simulink model "Spring2_Mass2_Damper2"  (R2019a)
settings: Solver=VariableStepAuto  StartTime=0.0  StopTime=100  RelTol=1e-3
values from neighbouring files (symbols this model uses):
  C1 = 1    [value.m]
  C2 = 1    [value.m]
  K1 = 1    [value.m]
  K2 = 1    [value.m]
  M1 = 1    [value.m]
  M2 = 1    [value.m]
settings Model: Creator=Takumi SHIOTA  LastModifiedBy=TakumiShiota

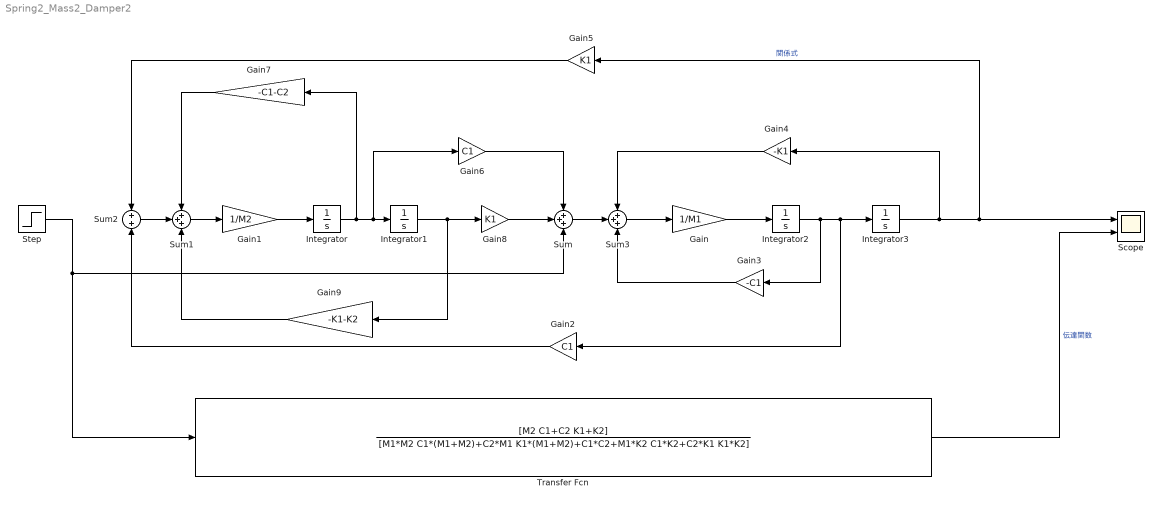
== system Spring2_Mass2_Damper2 ==
  Gain : Gain  Gain=1/M1
  Gain1 : Gain  Gain=1/M2
  Gain2 : Gain  Gain=C1
  Gain3 : Gain  Gain=-C1
  Gain4 : Gain  Gain=-K1
  Gain5 : Gain  Gain=K1
  Gain6 : Gain  Gain=C1
  Gain7 : Gain  Gain=-C1-C2
  Gain8 : Gain  Gain=K1
  Gain9 : Gain  Gain=-K1-K2
  Integrator{,1..3} (4 alike) : Integrator
  Scope : Scope  NumInputPorts=2
  Step : Step  SampleTime=0.0002
  Sum : Sum  Inputs=+++
  Sum1 : Sum  Inputs=+++
  Sum2 : Sum  Inputs=+|+
  Sum3 : Sum  Inputs=+++
  Transfer Fcn : TransferFcn  Numerator=[M2 C1+C2 K1+K2]  Denominator=[M1*M2 C1*(M1+M2)+C2*M1 K1*(M1+M2)+C1*C2+M1*K2 C1*K2+C2*K1 K1*K2]
  wires:
  Step/1 -> Sum/3, Transfer Fcn/1
  Transfer Fcn/1 -> Scope/2  "伝達関数"
  Sum2/1 -> Sum1/2
  Gain/1 -> Integrator2/1
  Integrator/1 -> Gain7/1, Gain6/1, Integrator1/1
  Integrator1/1 -> Gain9/1, Gain8/1
  Gain1/1 -> Integrator/1
  Sum3/1 -> Gain/1
  Integrator2/1 -> Gain3/1, Gain2/1, Integrator3/1
  Integrator3/1 -> Scope/1, Gain5/1, Gain4/1  "関係式"
  Gain6/1 -> Sum/1
  Gain4/1 -> Sum3/1
  Gain8/1 -> Sum/2
  Gain2/1 -> Sum2/2
  Gain3/1 -> Sum3/3
  Gain7/1 -> Sum1/1
  Gain5/1 -> Sum2/1
  Gain9/1 -> Sum1/3
  Sum/1 -> Sum3/2
  Sum1/1 -> Gain1/1
